simulink model "DOBC_whole_v2"  (R2022b)
settings: Solver=ode45  StartTime=0.0  StopTime=30  RelTol=1e-3  EnableMultiTasking=on
undefined symbols (not defined in the file): A_d, b_1, b_2, B_d, C_d, F_filter2_denom, F_filter2_num, F_filter_denom, F_filter_num, feedforward_switch, J_pend_1, J_pend_2, K_aug, K_g_1, K_g_2, K_int, K_m_1, K_m_2, K_pend_1, K_pend_2, K_SF, K_sin_1, K_sin_2, Kc, L_1, L_2, L_Pred, N, N1, N2, Np, Q_filter_denom, Q_filter_num, R_1, R_2, repetitive_switch, saturation, signal_switch, Tcomp, Ts, Tss, V_s_1, V_s_2
libraries: simulink x2, spsTriangleGeneratorLib x1
settings Model: Creator=Martin  LastModifiedBy=suzer
settings SolverCC: ZeroCrossControl=DisableAll  ZeroCrossAlgorithm=Adaptive  AlgebraicLoopSolver=TrustRegion
settings DataIOCC: ReturnWorkspaceOutputs=off
settings OptimizationCC: LifeSpan=inf
settings DebuggingCC: MaxConsecutiveZCsMsg=none  UnconnectedInputMsg=warning  UnconnectedOutputMsg=warning  UnconnectedLineMsg=warning  SFUnexpectedBacktrackingDiag=warning  SFNoUnconditionalDefaultTransitionDiag=warning  SFExecutionAtInitializationDiag=none  SFMachineParentedDataDiag=warning  ArithmeticOperatorsInVariantConditions=warning
settings ModelReferenceCC: EnableRefExpFcnMdlSchedulingChecks=on
settings SFSimCC: SimUseLocalCustomCode=off  CustomCodeUndefinedFunction=UseInterfaceOnly
settings RTWCC: RTWUseLocalCustomCode=off  DLArmComputeVersion=19.05
settings CodeAppCC: StateflowObjectComments=on
settings GRTTargetCC: TargetLangStandard=C89/C90 (ANSI)
settings ConfigComp: CovMetricSettings=dw  CovSaveCumulativeToWorkspaceVar=on  CovSaveSingleToWorkspaceVar=on  CovExternalEMLEnable=off

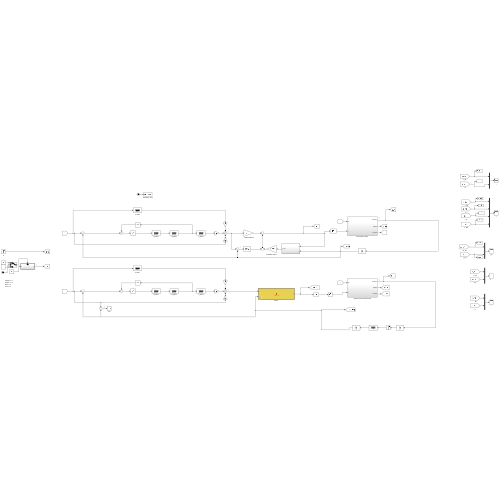
[thumbnail: Simulink's stored preview of the top-level diagram]
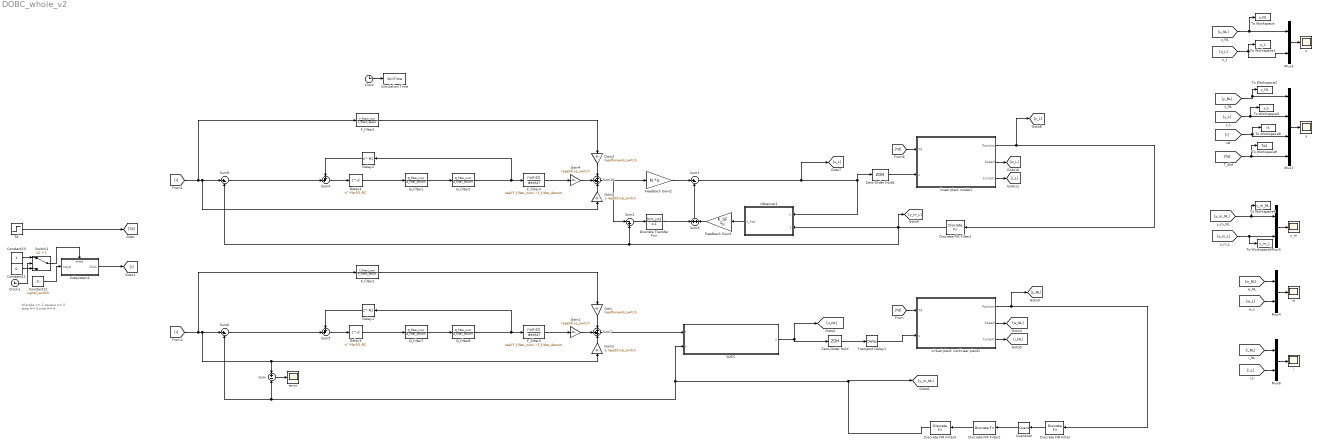
== system DOBC_whole_v2 ==
  note: triangle == 1
      | square == 2
      | step == 3
      | sine == 4
  Clock : Clock
  Clock1 : Clock
  Constant11 : Constant  Value=0
  Constant12 : Constant  Value=signal_switch
  Constant13 : Constant
  Delay1 : Delay  DelayLength=N1  SampleTime=Ts
  Delay2 : Delay  DelayLength=N1  SampleTime=Ts
  Delay3 : Delay  DelayLength=Np-N1-N2  SampleTime=Ts
  Delay4 : Delay  DelayLength=Np-N1-N2  SampleTime=Ts
  Discrete Transfer Fcn : DiscreteTransferFcn  Numerator=[0 K_int]  Denominator=[1 -1]  SampleTime=Ts
  Discrete FIR Filter : DiscreteFir  Coefficients=[1]  SampleTime=Tss
  Discrete FIR Filter1 : DiscreteFir  Coefficients=[1]  SampleTime=Ts
  Discrete FIR Filter2 : DiscreteFir  Coefficients=[0.25 0.25 0.25 0.25]
  Discrete FIR Filter3 : DiscreteFir  Coefficients=[1]  SampleTime=Ts
  F_filter1 : DiscreteFilter  Numerator=F_filter2_num  Denominator=F_filter2_denom  SampleTime=Ts
  F_filter2 : DiscreteFilter  Numerator=F_filter2_num  Denominator=F_filter2_denom  SampleTime=Ts
  F_filter3 : DiscreteFilter  Numerator=real(F_filter_num)  Denominator=F_filter_denom  SampleTime=Ts
  F_filter4 : DiscreteFilter  Numerator=real(F_filter_num)  Denominator=F_filter_denom  SampleTime=Ts
  Feedback Gain1 : Gain  Gain=K_SF  Multiplication=Matrix(K*u)
  Feedback Gain2 : Gain  Gain=N  Multiplication=Matrix(K*u)
  Gain : Gain  Gain=feedforward_switch
  Gain1 : Gain  Gain=repetitive_switch
  Gain2 : Gain  Gain=1-repetitive_switch
  Gain3 : Gain  Gain=feedforward_switch
  Gain4 : Gain  Gain=repetitive_switch
  Gain5 : Gain  Gain=1-repetitive_switch
  Mux1 : Mux
  Mux{3..6} (4 alike) : Mux  Inputs=2
  Observer1 : Subsystem
  Q_filter{1..2,7..8} (4 alike) : DiscreteFilter  Numerator=Q_filter_num  Denominator=Q_filter_denom  SampleTime=Ts
  Quantizer : Quantizer  QuantizationInterval=encoder_resolution
  SOFC : MATLAB Function  TreatAsAtomicUnit=on  mask{A=A_d, B=B_d, C=C_d, K=K_aug, L=L_Pred, N=N}
  Simulation Time : ToWorkspace  VariableName=SimTime  SampleTime=-1
  Subsystem1 : Subsystem
  Sum : Sum  Inputs=+|-
  Sum1 : Sum  Inputs=|+-
  Sum10 : Sum  Inputs=+++
  Sum2 : Sum  Inputs=|-+
  Sum3 : Sum  Inputs=+|+
  Sum4 : Sum  Inputs=++|
  Sum5 : Sum  Inputs=++|
  Sum6 : Sum  Inputs=|+-
  Sum7 : Sum  Inputs=+++
  Sum9 : Sum  Inputs=|+-
  Switch1 : Switch  Criteria=u2 > Threshold  Threshold=1  SaturateOnIntegerOverflow=off  InputSameDT=off
  Td : Step  Time=5  After=0.05  SampleTime=0
  To Workspace : ToWorkspace  VariableName=u_NL  SampleTime=Ts
  To Workspace1 : ToWorkspace  VariableName=u_L  SampleTime=Ts
  To Workspace2 : ToWorkspace  VariableName=y_NL  SampleTime=Ts
  To Workspace3 : ToWorkspace  VariableName=y_L  SampleTime=Ts
  To Workspace4 : ToWorkspace  VariableName=y_m_NL  SampleTime=Ts
  To Workspace5 : ToWorkspace  VariableName=y_m_L  SampleTime=Ts
  To Workspace8 : ToWorkspace  VariableName=r1  SampleTime=Ts
  To Workspace9 : ToWorkspace  VariableName=Td1  SampleTime=Ts
  Transport Delay1 : TransportDelay  DelayTime=Tcomp  BufferSize=4096  PadeOrder=2
  Zero-Order Hold : ZeroOrderHold  SampleTime=Ts
  Zero-Order Hold1 : ZeroOrderHold  SampleTime=Ts
  error : Scope
  i : Scope
  linear plant model1 : Subsystem
  u : Scope
  virtual plant: nonlinear plant1 : Subsystem
  "w\t" : Scope
  y : Scope
  y_m : Scope
  wires:
  Clock/1 -> Simulation Time/1
  virtual plant: nonlinear plant1/1(Position) -> [y_NL], Discrete FIR Filter/1
  virtual plant: nonlinear plant1/2(Speed) -> [w_NL]
  virtual plant: nonlinear plant1/3(Current) -> [i_NL]
  Quantizer/1 -> Discrete FIR Filter2/1
  Discrete FIR Filter/1 -> Quantizer/1
  SOFC/1(u) -> [u_NL], Zero-Order Hold/1
  [Td] -> virtual plant: nonlinear plant1/1(Td)
  Discrete FIR Filter2/1 -> Discrete FIR Filter3/1
  Discrete FIR Filter3/1 -> [y_m_NL], Sum/2, Sum6/2, SOFC/2(y)
  [u_NL] -> To Workspace/1, Mux3/1
  Mux3/1 -> u/1
  Mux1/1 -> y/1
  [y_NL] -> To Workspace2/1, Mux1/1
  [y_L] -> To Workspace3/1, Mux1/2
  Mux5/1 -> y_m/1
  [y_m_NL] -> To Workspace4/1, Mux5/1
  [y_m_L] -> To Workspace5/1, Mux5/2
  Mux4/1 -> "w\t"/1
  [w_NL] -> Mux4/1
  [w_L] -> Mux4/2
  Mux6/1 -> i/1
  [i_NL] -> Mux6/1
  [i_L] -> Mux6/2
  [u_L] -> To Workspace1/1, Mux3/2
  [r] -> To Workspace8/1, Mux1/3
  [Td] -> To Workspace9/1, Mux1/4
  Clock1/1 -> Switch1/2
  Constant13/1 -> Switch1/1
  Switch1/1 -> Subsystem1/Enable
  Constant11/1 -> Switch1/3
  Constant12/1 -> Subsystem1/1(Input)
  Sum5/1 -> Delay3/1
  Sum6/1 -> Sum5/2
  Zero-Order Hold/1 -> Transport Delay1/1
  Transport Delay1/1 -> virtual plant: nonlinear plant1/2(u)
  Sum7/1 -> SOFC/1(r)
  [r] -> Sum6/1, Sum/1, Gain2/1, F_filter1/1
  F_filter3/1 -> Gain1/1
  Sum10/1 -> Feedback Gain2/1, Sum2/1
  Zero-Order Hold1/1 -> linear plant model1/2(u)
  Observer1/1(x_hat) -> Feedback Gain1/1
  [Td] -> linear plant model1/1(Td)
  Sum3/1 -> Sum1/2
  linear plant model1/3(Current) -> [i_L]
  linear plant model1/1(Position) -> [y_L], Discrete FIR Filter1/1
  Sum1/1 -> [u_L], Observer1/1(u), Zero-Order Hold1/1
  linear plant model1/2(Speed) -> [w_L]
  Sum2/1 -> Discrete Transfer Fcn/1
  Discrete Transfer Fcn/1 -> Sum3/1
  Feedback Gain2/1 -> Sum1/1
  Feedback Gain1/1 -> Sum3/2
  F_filter1/1 -> Gain/1
  Delay3/1 -> Q_filter7/1
  Delay1/1 -> Sum5/1
  Q_filter7/1 -> Q_filter8/1
  Q_filter8/1 -> Delay1/1, F_filter3/1
  Subsystem1/1(Out1) -> [r]
  Gain/1 -> Sum7/1
  Gain1/1 -> Sum7/2
  Gain2/1 -> Sum7/3
  Td/1 -> [Td]
  Discrete FIR Filter1/1 -> Sum2/2, Sum9/2, Observer1/2(y), [y_m_L]
  Q_filter2/1 -> Delay2/1, F_filter4/1
  Delay2/1 -> Sum4/1
  Q_filter1/1 -> Q_filter2/1
  F_filter2/1 -> Gain3/1
  [r] -> Sum9/1, Gain5/1, F_filter2/1
  Sum9/1 -> Sum4/2
  Sum4/1 -> Delay4/1
  F_filter4/1 -> Gain4/1
  Delay4/1 -> Q_filter1/1
  Gain5/1 -> Sum10/3
  Gain4/1 -> Sum10/2
  Gain3/1 -> Sum10/1
  Sum/1 -> error/1

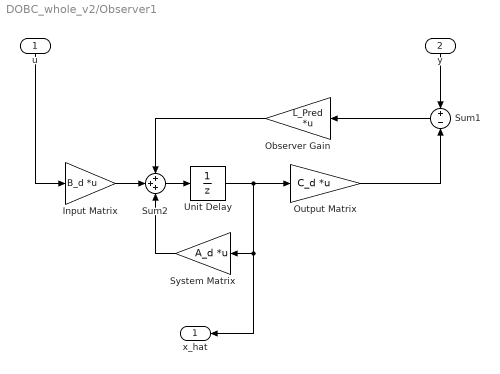
== system DOBC_whole_v2/Observer1 ==
  u : Inport
  y : Inport  Port=2
  Input Matrix : Gain  Gain=B_d  Multiplication=Matrix(K*u)
  Observer Gain : Gain  Gain=L_Pred  Multiplication=Matrix(K*u)
  Output Matrix : Gain  Gain=C_d  Multiplication=Matrix(K*u)
  Sum1 : Sum  Inputs=+|-
  Sum2 : Sum  Inputs=+++
  System Matrix : Gain  Gain=A_d  Multiplication=Matrix(K*u)
  Unit Delay : UnitDelay  SampleTime=Ts  HasFrameUpgradeWarning=on
  x_hat : Outport
  wires:
  Sum1/1 -> Observer Gain/1
  System Matrix/1 -> Sum2/3
  Sum2/1 -> Unit Delay/1
  Output Matrix/1 -> Sum1/2
  Input Matrix/1 -> Sum2/2
  Observer Gain/1 -> Sum2/1
  u/1 -> Input Matrix/1
  Unit Delay/1 -> x_hat/1, System Matrix/1, Output Matrix/1
  y/1 -> Sum1/1

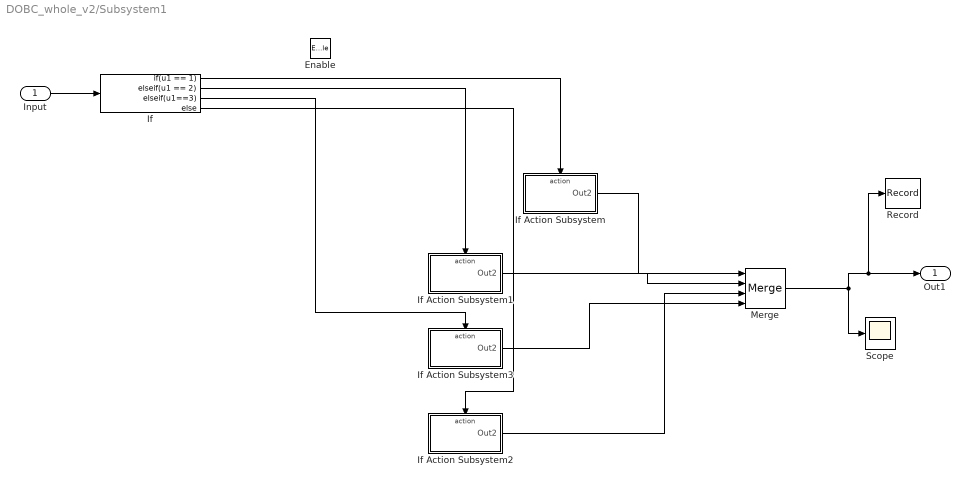
== system DOBC_whole_v2/Subsystem1 ==
  Input : Inport
  Enable : EnablePort
  If : If  IfExpression=u1 == 1  ElseIfExpressions=u1 == 2,u1==3
  If Action Subsystem : Subsystem  TreatAsAtomicUnit=on
  If Action Subsystem1 : Subsystem  TreatAsAtomicUnit=on
  If Action Subsystem2 : Subsystem  TreatAsAtomicUnit=on
  If Action Subsystem3 : Subsystem  TreatAsAtomicUnit=on
  Merge : Merge  Inputs=4
  Record : Record  FileSettingsInternal="{\"entries\":[{\"content\":{\"excelSettings\":{\"content\":{},\"type\":\"Streamout.ExcelSettings\"}},\"type\":\"Streamout.FileSettingStorage\",\"uuid\":\"6662721f-2ff1-4169-acb3-3573d75459ff\"}],\"packageUris\":[\"http://schema.mathworks.com/mf0/streamout_blocks/R2020a\"],\"version\":\"1.0\"}"  Layout=[1 1]  SignalsInternal="{\"entries\":[{\"content\":{\"signals\":[{\"content\":{\"blockPath\":[\"DOBC_whole_v2/Subsystem1/Record\"],\"channel\":[],\"dimensions\":[1],\"domain\":\"DOBC_whole_v2/Subsystem1/Record\",\"lineColor\":\"#22b573\",\"plots\":[1],\"port\":1,\"sid\":[],\"signalID\":406,\"signalName\":\"Merge\"},\"type\":\"RecordBlkView.Signal\",\"uuid\":\"65e2031a-14ab-4fd6-b67b-1a04d588579a\"}]},\"type\":\"RecordBlkView.InputSignals\",\"uuid\":\"f925c740-60ff-405b-b294-f11fa5d0c0e1\"}],\"packageUris\":[\"http://schema.mathworks.com/mf0/streamout_blocks/R2020a\"],\"version\":\"1.0\"}"
  Scope : Scope
  Out1 : Outport
  wires:
  If/1 -> If Action Subsystem/Action
  Merge/1 -> Out1/1, Record/1, Scope/1
  If Action Subsystem2/1(Out2) -> Merge/3
  If Action Subsystem1/1(Out2) -> Merge/2
  If Action Subsystem/1(Out2) -> Merge/1
  If/4 -> If Action Subsystem2/Action
  If/2 -> If Action Subsystem1/Action
  Input/1 -> If/1
  If/3 -> If Action Subsystem3/Action
  If Action Subsystem3/1(Out2) -> Merge/4

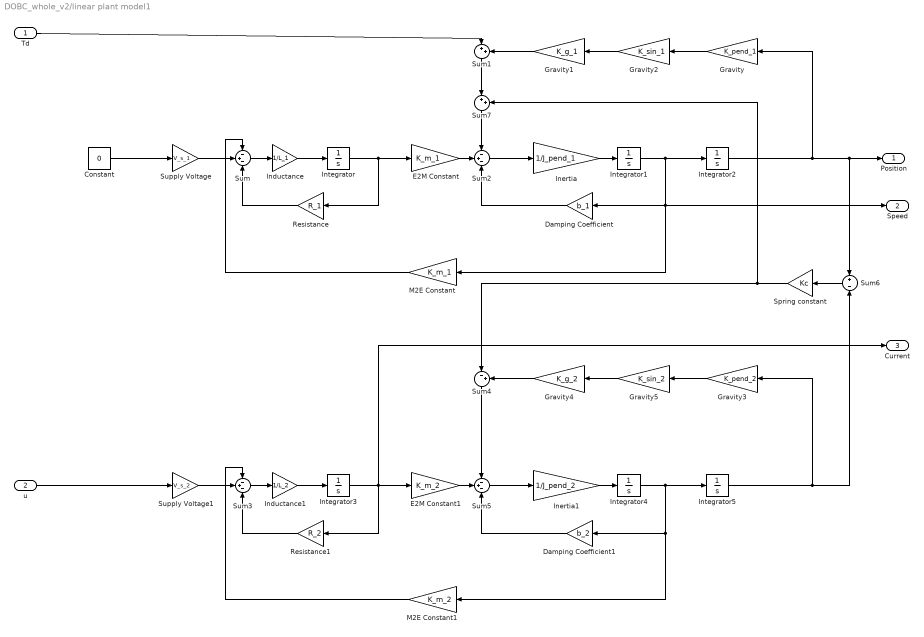
== system DOBC_whole_v2/linear plant model1 ==
  Td : Inport
  u : Inport  Port=2
  Constant : Constant  Value=0
  Damping Coefficient : Gain  Gain=b_1
  Damping Coefficient1 : Gain  Gain=b_2
  E2M Constant : Gain  Gain=K_m_1
  E2M Constant1 : Gain  Gain=K_m_2
  Gravity : Gain  Gain=K_pend_1
  Gravity1 : Gain  Gain=K_g_1
  Gravity2 : Gain  Gain=K_sin_1
  Gravity3 : Gain  Gain=K_pend_2
  Gravity4 : Gain  Gain=K_g_2
  Gravity5 : Gain  Gain=K_sin_2
  Inductance : Gain  Gain=1/L_1
  Inductance1 : Gain  Gain=1/L_2
  Inertia : Gain  Gain=1/J_pend_1
  Inertia1 : Gain  Gain=1/J_pend_2
  Integrator{,1..5} (6 alike) : Integrator
  M2E Constant : Gain  Gain=K_m_1
  M2E Constant1 : Gain  Gain=K_m_2
  Resistance : Gain  Gain=R_1
  Resistance1 : Gain  Gain=R_2
  Spring constant : Gain  Gain=Kc
  Sum{,2..3,5} (4 alike) : Sum  Inputs=-+-
  Sum1 : Sum  Inputs=|++
  Sum4 : Sum  Inputs=|-+
  Sum6 : Sum  Inputs=+|-
  Sum7 : Sum  Inputs=|++
  Supply Voltage : Gain  Gain=V_s_1
  Supply Voltage1 : Gain  Gain=V_s_2
  Position : Outport
  Speed : Outport  Port=2
  Current : Outport  Port=3
  wires:
  Damping Coefficient/1 -> Sum2/3
  Gravity/1 -> Gravity2/1
  Integrator/1 -> E2M Constant/1, Resistance/1
  Integrator1/1 -> Damping Coefficient/1, Speed/1, M2E Constant/1, Integrator2/1
  Resistance/1 -> Sum/3
  Sum/1 -> Inductance/1
  Inductance/1 -> Integrator/1
  Supply Voltage/1 -> Sum/2
  M2E Constant/1 -> Sum/1
  Sum2/1 -> Inertia/1
  Inertia/1 -> Integrator1/1
  E2M Constant/1 -> Sum2/2
  Td/1 -> Sum1/1
  Integrator2/1 -> Gravity/1, Sum6/1, Position/1
  Gravity1/1 -> Sum1/2
  Gravity2/1 -> Gravity1/1
  Sum6/1 -> Spring constant/1
  Gravity5/1 -> Gravity4/1
  Gravity4/1 -> Sum4/2
  Integrator5/1 -> Sum6/2, Gravity3/1
  u/1 -> Supply Voltage1/1
  E2M Constant1/1 -> Sum5/2
  Inertia1/1 -> Integrator4/1
  Sum5/1 -> Inertia1/1
  M2E Constant1/1 -> Sum3/1
  Supply Voltage1/1 -> Sum3/2
  Inductance1/1 -> Integrator3/1
  Sum3/1 -> Inductance1/1
  Resistance1/1 -> Sum3/3
  Integrator4/1 -> Integrator5/1, M2E Constant1/1, Damping Coefficient1/1
  Integrator3/1 -> Current/1, Resistance1/1, E2M Constant1/1
  Gravity3/1 -> Gravity5/1
  Sum4/1 -> Sum5/1
  Damping Coefficient1/1 -> Sum5/3
  Sum1/1 -> Sum7/1
  Sum7/1 -> Sum2/1
  Spring constant/1 -> Sum4/1, Sum7/2
  Constant/1 -> Supply Voltage/1

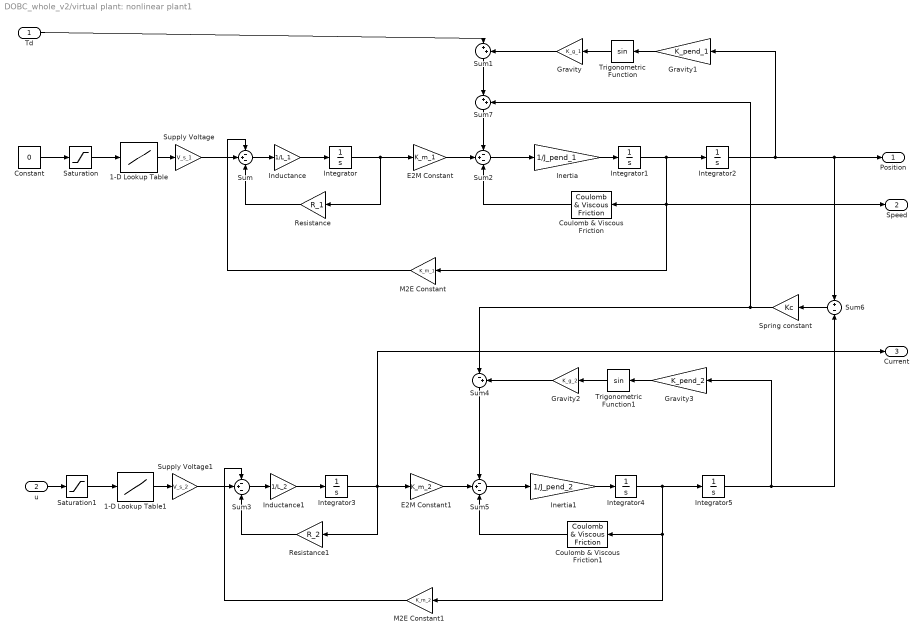
== system DOBC_whole_v2/virtual plant: nonlinear plant1 ==
  Td : Inport
  u : Inport  Port=2
  1-D Lookup Table : Lookup_n-D  NumberOfTableDimensions=1  BreakpointsForDimension1=[-1,-0.96,-0.1,-0.06,-0.04,0,0.04,0.06,0.1,0.96,1]  Table=[-10.8,-10.8,-2,-1,-0,0,0,1,2,10.8,10.8]/V_s_1  InternalRulePriority=Speed  RndMeth=Simplest
  1-D Lookup Table1 : Lookup_n-D  NumberOfTableDimensions=1  BreakpointsForDimension1=[-1,-0.96,-0.1,-0.06,-0.04,0,0.04,0.06,0.1,0.96,1]  Table=[-10.8,-10.8,-2,-1,-0,0,0,1,2,10.8,10.8]/V_s_2  InternalRulePriority=Speed  RndMeth=Simplest
  Constant : Constant  Value=0
  Coulomb & Viscous Friction : simulink/Discontinuities/Coulomb & Viscous Friction  offset=Friction_static  gain=b_1
  Coulomb & Viscous Friction1 : simulink/Discontinuities/Coulomb & Viscous Friction  offset=Friction_static  gain=b_1
  E2M Constant : Gain  Gain=K_m_1
  E2M Constant1 : Gain  Gain=K_m_2
  Gravity : Gain  Gain=K_g_1
  Gravity1 : Gain  Gain=K_pend_1
  Gravity2 : Gain  Gain=K_g_2
  Gravity3 : Gain  Gain=K_pend_2
  Inductance : Gain  Gain=1/L_1
  Inductance1 : Gain  Gain=1/L_2
  Inertia : Gain  Gain=1/J_pend_1
  Inertia1 : Gain  Gain=1/J_pend_2
  Integrator{,1..5} (6 alike) : Integrator
  M2E Constant : Gain  Gain=K_m_1
  M2E Constant1 : Gain  Gain=K_m_2
  Resistance : Gain  Gain=R_1
  Resistance1 : Gain  Gain=R_2
  Saturation : Saturate  UpperLimit=saturation  LowerLimit=-saturation
  Saturation1 : Saturate  UpperLimit=saturation  LowerLimit=-saturation
  Spring constant : Gain  Gain=Kc
  Sum{,2..3,5} (4 alike) : Sum  Inputs=-+-
  Sum1 : Sum  Inputs=|++
  Sum4 : Sum  Inputs=|-+
  Sum6 : Sum  Inputs=+|-
  Sum7 : Sum  Inputs=|++
  Supply Voltage : Gain  Gain=V_s_1
  Supply Voltage1 : Gain  Gain=V_s_2
  Trigonometric Function : Trigonometry
  Trigonometric Function1 : Trigonometry
  Position : Outport
  Speed : Outport  Port=2
  Current : Outport  Port=3
  wires:
  Coulomb & Viscous Friction/1 -> Sum2/3
  Gravity/1 -> Sum1/2
  Integrator/1 -> E2M Constant/1, Resistance/1
  Integrator1/1 -> Coulomb & Viscous Friction/1, Speed/1, M2E Constant/1, Integrator2/1
  Resistance/1 -> Sum/3
  Trigonometric Function/1 -> Gravity/1
  Sum/1 -> Inductance/1
  Inductance/1 -> Integrator/1
  Supply Voltage/1 -> Sum/2
  M2E Constant/1 -> Sum/1
  Sum2/1 -> Inertia/1
  Inertia/1 -> Integrator1/1
  Saturation/1 -> 1-D Lookup Table/1
  E2M Constant/1 -> Sum2/2
  1-D Lookup Table/1 -> Supply Voltage/1
  Td/1 -> Sum1/1
  Gravity1/1 -> Trigonometric Function/1
  Sum4/1 -> Sum5/1
  Gravity3/1 -> Trigonometric Function1/1
  1-D Lookup Table1/1 -> Supply Voltage1/1
  E2M Constant1/1 -> Sum5/2
  Saturation1/1 -> 1-D Lookup Table1/1
  Inertia1/1 -> Integrator4/1
  Sum5/1 -> Inertia1/1
  M2E Constant1/1 -> Sum3/1
  Supply Voltage1/1 -> Sum3/2
  Inductance1/1 -> Integrator3/1
  Sum3/1 -> Inductance1/1
  Trigonometric Function1/1 -> Gravity2/1
  Resistance1/1 -> Sum3/3
  Integrator4/1 -> Integrator5/1, M2E Constant1/1, Coulomb & Viscous Friction1/1
  Integrator3/1 -> Current/1, Resistance1/1, E2M Constant1/1
  Gravity2/1 -> Sum4/2
  Coulomb & Viscous Friction1/1 -> Sum5/3
  Sum6/1 -> Spring constant/1
  u/1 -> Saturation1/1
  Sum1/1 -> Sum7/1
  Sum7/1 -> Sum2/1
  Spring constant/1 -> Sum4/1, Sum7/2
  Integrator2/1 -> Sum6/1, Position/1, Gravity1/1
  Integrator5/1 -> Sum6/2, Gravity3/1
  Constant/1 -> Saturation/1

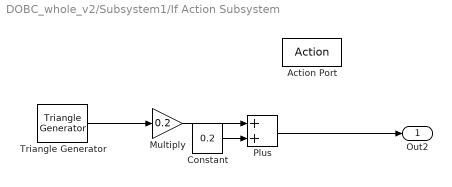
== system DOBC_whole_v2/Subsystem1/If Action Subsystem ==
  Action Port : ActionPort  ActionPortLabel=if(u1 == 1)
  Constant : Constant  Value=0.2
  Multiply : Gain  Gain=0.2
  Plus : Sum
  Triangle Generator : spsTriangleGeneratorLib/Triangle Generator  Freq=d_hz  Phase=0  Ts=Ts
  Out2 : Outport
  wires:
  Constant/1 -> Plus/2
  Plus/1 -> Out2/1
  Triangle Generator/1 -> Multiply/1
  Multiply/1 -> Plus/1

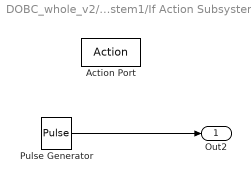
== system DOBC_whole_v2/Subsystem1/If Action Subsystem1 ==
  Action Port : ActionPort  ActionPortLabel=elseif(u1 == 2)
  Pulse Generator : DiscretePulseGenerator  Amplitude=0.4  Period=1/d_hz/Ts  PulseWidth=1/d_hz/2/Ts  SampleTime=Ts
  Out2 : Outport
  wires:
  Pulse Generator/1 -> Out2/1

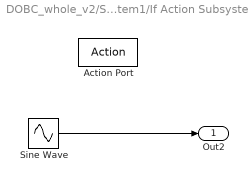
== system DOBC_whole_v2/Subsystem1/If Action Subsystem2 ==
  Action Port : ActionPort  ActionPortLabel=else
  Sine Wave : Sin  SineType=Sample based  Amplitude=0.2  Bias=0.2  Samples=1/d_hz/Ts  SampleTime=Ts  Offset=0.75*1/d_hz/Ts
  Out2 : Outport
  wires:
  Sine Wave/1 -> Out2/1

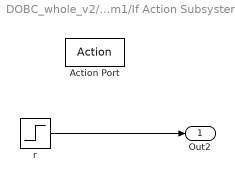
== system DOBC_whole_v2/Subsystem1/If Action Subsystem3 ==
  Action Port : ActionPort  ActionPortLabel=elseif(u1==3)
  r : Step  After=pi  SampleTime=Ts
  Out2 : Outport
  wires:
  r/1 -> Out2/1

== matlab function DOBC_whole_v2/SOFC ==
  data: r input; u output; y input; A parameter; B parameter; C parameter; K parameter; L parameter; N parameter
function u = controller(r,y,A, B, C, K, L, N)

persistent xhat xint;  %memory for the state

  if isempty(xhat)  %local variable initialization
      n=size(L,1);
        xhat=zeros(n,1); 
      m = size(K,2)-n;
        xint=zeros(m,1);  
  end
xaug=[xhat; xint]; %Augmented state include the state for the integrator
%u = -K*xaug+N*r; %Control computation with integral action 
u_unsat = -K*xaug+N*r; %Control computation with integral action 
u= sign(u_unsat)*min(1,abs(u_unsat));
%DAC(u) send out control here to minimize computation delay
%Update the next state next
xhat = (A-L*C)*xhat + B*u + L*y;
xint = xint+ y-r;
